simulink model "WS_17_Nils_Bestehorn_modell_ABCD"  (R2021b)
settings: Solver=VariableStepAuto  StartTime=0.0  StopTime=20.0  RelTol=1e-3
values from neighbouring files (symbols this model uses):
  A = [0 0 1 0 0 ... (first row only)    [WS_17_Nils_Bestehorn_mfile.m]
  B = [0; 0; c1/m1; cp/m2; cp/dp]    [WS_17_Nils_Bestehorn_mfile.m]
  C = [c2 -c2 0 0 0 ... (first row only)    [WS_17_Nils_Bestehorn_mfile.m]
  D = [0;0]    [WS_17_Nils_Bestehorn_mfile.m]
  zh = 10*10^-2    (= 0.1)    [WS_17_Nils_Bestehorn_mfile.m]
undefined symbols (not defined in the file or in its folder): sigbuilder_block
libraries: simulink x1
settings Model: Creator=nilsb  LastModifiedBy=nilsb

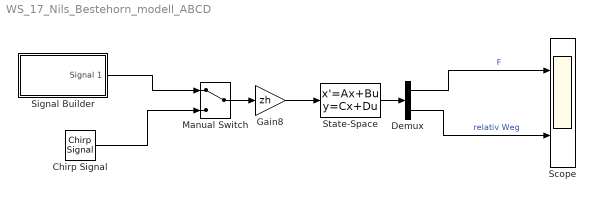
== system WS_17_Nils_Bestehorn_modell_ABCD ==
  Chirp Signal : simulink/Sources/Chirp Signal  f1=0.01  T=20  f2=20
  Demux : Demux  Outputs=2
  Gain8 : Gain  Gain=zh
  Manual Switch : ManualSwitch
  Scope : Scope  NumInputPorts=2
  Signal Builder : Subsystem  Tag=STV Subsys  LoadFcn=sigbuilder_block('load');  StartFcn=sigbuilder_block('start');  StopFcn=sigbuilder_block('stop');  ClipboardFcn=sigbuilder_block('clipboard');  mask(Sigbuilder block){tuvar=[0:10]}
      mask help: Simulink:masks:SigbuilderBlock_MD
      mask init:
      | if ~strcmp(get_param(bdroot(gcbh),'SimulationStatus'),'stopped') tuvar = sigbuilder_block('maskInit'); end
      settings: CopyFcn=sigbuilder_block('copy');  DeleteFcn=sigbuilder_block('delete');  ModelCloseFcn=sigbuilder_block('modelClose');  PreSaveFcn=sigbuilder_block('preSave');  PauseFcn=sigbuilder_block('pause');  ContinueFcn=sigbuilder_block('continue');  NameChangeFcn=sigbuilder_block('namechange');  OpenFcn=sigbuilder_block('open',[437.6 199.2 550.4 400 ]);  CloseFcn=sigbuilder_block('close');
      mask Display: plot(0, 0, 100, 100,[2, 2, 32, 32, 2], [68, 8, 8, 68, 68],[32, 2], [38, 38], [32, 19, 2],[53, 60, 44], [32, 17, 17, 2],[16, 16, 31, 31]);txt = getActiveGroup(gcbh);text(2, 100, txt,'verticalAlignment', 'top');
  State-Space : StateSpace  A=A  B=B  C=C  D=D  InitialCondition=0
  wires:
  Gain8/1 -> State-Space/1
  State-Space/1 -> Demux/1
  Demux/1 -> Scope/1  "F"
  Demux/2 -> Scope/2  "relativ Weg"
  Manual Switch/1 -> Gain8/1
  Signal Builder/1(Signal 1) -> Manual Switch/1
  Chirp Signal/1 -> Manual Switch/2

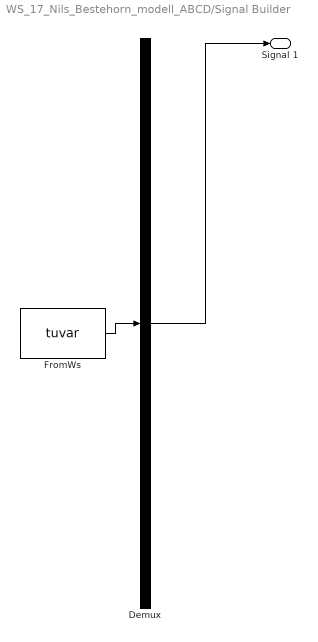
== system WS_17_Nils_Bestehorn_modell_ABCD/Signal Builder ==
  Demux : Demux  Tag=STV Demux  Outputs=1
      settings: DisplayOption=none
  FromWs : FromWorkspace  Tag=STV FromWs  VariableName=tuvar
      SigBuilderData=|
      | common.afterFinalStr = 'Extrapolate'
      | common.sampleTime = 0
      | dataSet.timeRange = [0 4]
      | dataSet.name = 'Group 1'
      | sbobj.Groups.Name = 'Group 1'
      | sbobj.Groups.Signals.Name = 'Signal 1'
      | sbobj.Groups.Signals.XData = [0 0.25 1.9 2 4]
      | sbobj.Groups.Signals.YData = [0 1 1 0 0]
      | sbobj.Groups.TimeRange = [0 4]
  Signal 1 : Outport  Tag=STV Outport
  wires:
  Demux/1 -> Signal 1/1
  FromWs/1 -> Demux/1
